simulink model "ukol_5_model"  (R2017a)
settings: Solver=VariableStepAuto  StartTime=0.0  StopTime=30  MaxStep=1e-2  RelTol=1e-3
values from neighbouring files (symbols this model uses):
  A = [0 1; -1.44 -0.36]    [ukol_5_script.m]
  B = [0; 1]    [ukol_5_script.m]
  C = [7.2 0; 0 7.2]    [ukol_5_script.m]    (also in ukol_8_script.m = C_1; ukol_9_script.m)
  D = [0; 0]    [ukol_5_script.m]    (also in ukol_8_script.m = 0; ukol_9_script.m)
  k1 = 0.982    [ukol_5_script.m]    (also in ukol_9_script.m)
  k1_2 = 6.645    [ukol_5_script.m]
  k2 = 1.8188    [ukol_5_script.m]    (also in ukol_9_script.m)
  k2_2 = 3.083    [ukol_5_script.m]
  kI = 3.767    [ukol_5_script.m]
  korekcni_zesileni = 1/0.846    (= 1.18203309693)    [ukol_5_script.m]
settings Model: Creator=tomas  LastModifiedBy=tomas

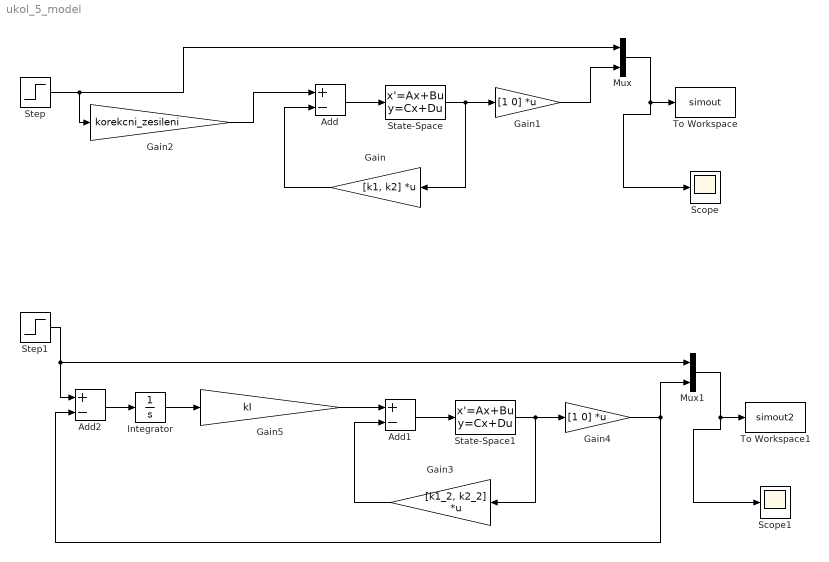
== system ukol_5_model ==
  Add : Sum  Inputs=+-
  Add1 : Sum  Inputs=+-
  Add2 : Sum  Inputs=+-
  Gain : Gain  Gain=[k1, k2]  Multiplication=Matrix(K*u)
  Gain1 : Gain  Gain=[1 0]  Multiplication=Matrix(K*u)
  Gain2 : Gain  Gain=korekcni_zesileni
  Gain3 : Gain  Gain=[k1_2, k2_2]  Multiplication=Matrix(K*u)
  Gain4 : Gain  Gain=[1 0]  Multiplication=Matrix(K*u)
  Gain5 : Gain  Gain=kI
  Integrator : Integrator
  Mux : Mux  Inputs=2
  Mux1 : Mux  Inputs=2
  Scope : Scope
  Scope1 : Scope
  State-Space : StateSpace  A=A  B=B  C=C  D=D  X0=0
  State-Space1 : StateSpace  A=A  B=B  C=C  D=D  X0=0
  Step : Step  SampleTime=0
  Step1 : Step  SampleTime=0
  To Workspace : ToWorkspace  VariableName=simout  SaveFormat=Timeseries  SampleTime=-1
  To Workspace1 : ToWorkspace  VariableName=simout2  SaveFormat=Timeseries  SampleTime=-1
  wires:
  State-Space/1 -> Gain/1, Gain1/1
  Add/1 -> State-Space/1
  Gain/1 -> Add/2
  Gain1/1 -> Mux/2
  Mux/1 -> Scope/1, To Workspace/1
  Step/1 -> Gain2/1, Mux/1
  Gain2/1 -> Add/1
  Gain5/1 -> Add1/1
  Gain4/1 -> Add2/2, Mux1/2
  State-Space1/1 -> Gain3/1, Gain4/1
  Add1/1 -> State-Space1/1
  Mux1/1 -> Scope1/1, To Workspace1/1
  Gain3/1 -> Add1/2
  Integrator/1 -> Gain5/1
  Add2/1 -> Integrator/1
  Step1/1 -> Mux1/1, Add2/1
